simulink model "ControllerForOriginSensordata"  (R2017a)
settings: Solver=FixedStepAuto  StartTime=0.0  StopTime=10  FixedStep=dt  RelTol=1e-3
values from neighbouring files (symbols this model uses):
  dt = dtFC    [evalOriginSensordata.m]    (also in startControllerNL.m = 0.01)
  H_Drone = zeros(5,12)    [evalOriginSensordata.m]    (also in startControllerNL.m)
  H_TWB = zeros(3,12)    [evalOriginSensordata.m]    (also in startControllerNL.m)
  k1 = a    (= 1)    [evalOriginSensordata.m]    (also in startControllerNL.m)
  k10 = a    (= 1)    [evalOriginSensordata.m]    (also in startControllerNL.m)
  k11 = a    (= 1)    [evalOriginSensordata.m]    (also in startControllerNL.m)
  k12 = a    (= 1)    [evalOriginSensordata.m]    (also in startControllerNL.m)
  k2 = a    (= 1)    [evalOriginSensordata.m]    (also in startControllerNL.m)
  k3 = a    (= 1)    [evalOriginSensordata.m]    (also in startControllerNL.m)
  k4 = a    (= 1)    [evalOriginSensordata.m]    (also in startControllerNL.m)
  k5 = a    (= 1)    [evalOriginSensordata.m]    (also in startControllerNL.m)
  k6 = a    (= 1)    [evalOriginSensordata.m]    (also in startControllerNL.m)
  k7 = a    (= 1)    [evalOriginSensordata.m]    (also in startControllerNL.m)
  k8 = a    (= 1)    [evalOriginSensordata.m]    (also in startControllerNL.m)
  k9 = a    (= 1)    [evalOriginSensordata.m]    (also in startControllerNL.m)
  kd1 = d    (= 10)    [evalOriginSensordata.m]    (also in startControllerNL.m)
  kd2 = d    (= 10)    [evalOriginSensordata.m]    (also in startControllerNL.m)
  kd3 = d    (= 10)    [evalOriginSensordata.m]    (also in startControllerNL.m)
  kd4 = d    (= 10)    [evalOriginSensordata.m]    (also in startControllerNL.m)
  kp1 = p    (= 5)    [evalOriginSensordata.m]    (also in startControllerNL.m)
  kp2 = p    (= 5)    [evalOriginSensordata.m]    (also in startControllerNL.m)
  kp3 = p    (= 5)    [evalOriginSensordata.m]    (also in startControllerNL.m)
  kp4 = p    (= 5)    [evalOriginSensordata.m]    (also in startControllerNL.m)
  x_d = [sensordataTWB(end,[2:4]), 0]    [evalOriginSensordata.m]    (also in startControllerNL.m = [0 0 8 0])
libraries: simulink x2, sharedTrackingLibrary x1
settings Model: Creator=Schalker  LastModifiedBy=Schalker

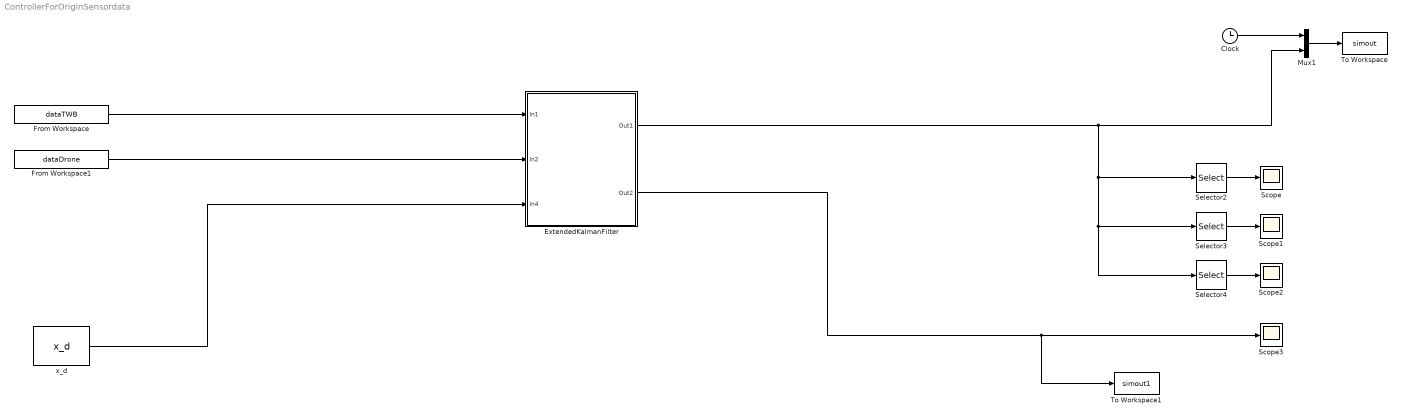
== system ControllerForOriginSensordata ==
  Clock : Clock
  "ExtendedKalmanFilter " : Subsystem
  From Workspace : FromWorkspace  VariableName=dataTWB  OutDataTypeStr=double  SampleTime=0
  From Workspace1 : FromWorkspace  VariableName=dataDrone  SampleTime=0
  Mux1 : Mux  Inputs=2
  Scope{,1..3} (4 alike) : Scope
  Selector2 : Selector  InputPortWidth=12  IndexOptions=Index vector (dialog)  Indices=1  OutputSizes=1
  Selector3 : Selector  InputPortWidth=12  IndexOptions=Index vector (dialog)  Indices=2  OutputSizes=1
  Selector4 : Selector  InputPortWidth=12  IndexOptions=Index vector (dialog)  Indices=3  OutputSizes=1
  To Workspace : ToWorkspace  VariableName=simout  SampleTime=-1
      settings: Save2DSignal=2-D array (concatenate along first dimension)
  To Workspace1 : ToWorkspace  VariableName=simout1  SampleTime=-1
      settings: Save2DSignal=2-D array (concatenate along first dimension)
  "x_d " : Constant  Value=x_d
  wires:
  Selector2/1 -> Scope/1
  Selector3/1 -> Scope1/1
  "ExtendedKalmanFilter "/1(Out1) -> Mux1/2, Selector4/1, Selector3/1, Selector2/1
  From Workspace/1 -> "ExtendedKalmanFilter "/1(In1)
  From Workspace1/1 -> "ExtendedKalmanFilter "/2(In2)
  "x_d "/1 -> "ExtendedKalmanFilter "/3(In4)
  "ExtendedKalmanFilter "/2(Out2) -> To Workspace1/1, Scope3/1
  Mux1/1 -> To Workspace/1
  Clock/1 -> Mux1/1
  Selector4/1 -> Scope2/1

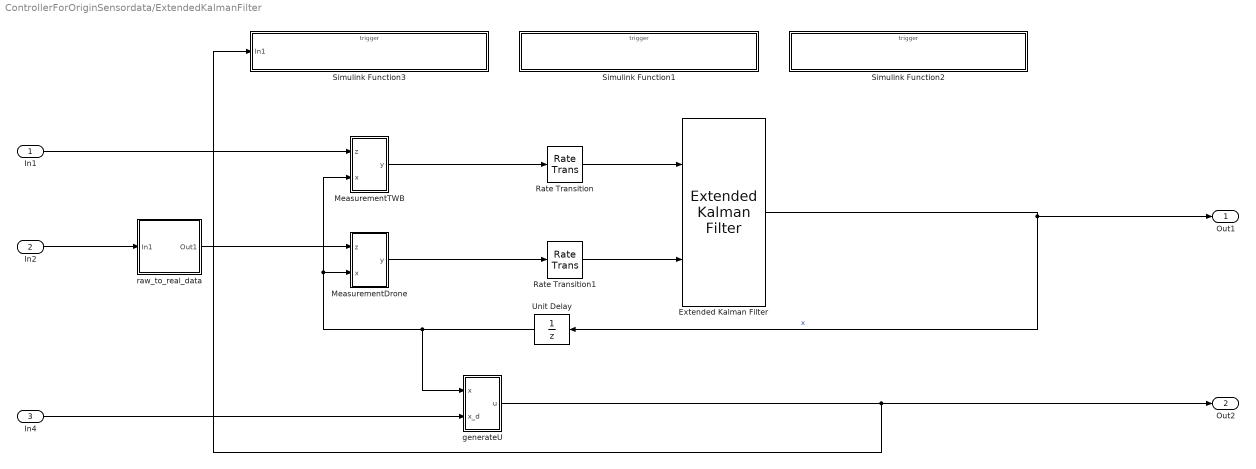
== system ControllerForOriginSensordata/ExtendedKalmanFilter  ==
  In1 : Inport
  In2 : Inport  Port=2
  In4 : Inport  Port=3
  Extended Kalman Filter : sharedTrackingLibrary/Extended Kalman Filter  StateTransitionFcn=stateTransitionFcn  HasStateTransitionJacobianFcn=off  HasAdditiveProcessNoise=Additive  ProcessNoise=processNoiseCovariance  HasTimeVaryingProcessNoise=off  HasStateTransitionFcnExtraArgument=0  InitialState=initialState  InitialStateCovariance=10  MeasurementFcn1=measurementTWBFcn  HasMeasurementJacobianFcn1=off  HasMeasurementEnablePort1=off  HasAdditiveMeasurementNoise1=Additive  MeasurementNoise1=measurementNoiseCovarianceTWB  HasTimeVaryingMeasurementNoise1=off  HasMeasurementFcnExtraArgument1=0  MeasurementFcn2=measurementDroneFcn  HasMeasurementJacobianFcn2=off  HasMeasurementEnablePort2=off  HasAdditiveMeasurementNoise2=Additive  MeasurementNoise2=measurementNoiseCovarianceDrone  HasTimeVaryingMeasurementNoise2=off  HasMeasurementFcnExtraArgument2=0  MeasurementFcn3=myMeasurementFcn  HasMeasurementJacobianFcn3=off  HasMeasurementEnablePort3=off  HasAdditiveMeasurementNoise3=Additive  MeasurementNoise3=1  HasTimeVaryingMeasurementNoise3=off  HasMeasurementFcnExtraArgument3=0  MeasurementFcn4=myMeasurementFcn  HasMeasurementJacobianFcn4=off  HasMeasurementEnablePort4=off  HasAdditiveMeasurementNoise4=Additive  MeasurementNoise4=1  HasTimeVaryingMeasurementNoise4=off  HasMeasurementFcnExtraArgument4=0  MeasurementFcn5=myMeasurementFcn  HasMeasurementJacobianFcn5=off  HasMeasurementEnablePort5=off  HasAdditiveMeasurementNoise5=Additive  MeasurementNoise5=1  HasTimeVaryingMeasurementNoise5=off  HasMeasurementFcnExtraArgument5=0  EnableMultirate=on  StateTransitionFcnSampleTime=dt  MeasurementFcn1SampleTime=dt  MeasurementFcn2SampleTime=dt  MeasurementFcn3SampleTime=1  MeasurementFcn4SampleTime=1  MeasurementFcn5SampleTime=1  UseCurrentEstimator=on  OutputStateCovariance=off  DataType=double  SampleTime=1  NumberOfMeasurements=2
  MeasurementDrone : Subsystem
  MeasurementTWB : Subsystem
  Rate Transition : RateTransition
  Rate Transition1 : RateTransition
  Simulink Function1 : Subsystem  TreatAsAtomicUnit=on
  Simulink Function2 : Subsystem  TreatAsAtomicUnit=on
  Simulink Function3 : Subsystem  TreatAsAtomicUnit=on
  Unit Delay : UnitDelay  SampleTime=-1
  generateU : Subsystem
  raw_to_real_data : Subsystem
  Out1 : Outport
  Out2 : Outport  Port=2
  wires:
  In1/1 -> MeasurementTWB/1(z)
  In4/1 -> generateU/2("x_d ")
  Extended Kalman Filter/1 -> Unit Delay/1, Out1/1  "x"
  MeasurementDrone/1(y) -> Rate Transition1/1
  Rate Transition1/1 -> Extended Kalman Filter/2
  In2/1 -> raw_to_real_data/1(In1)
  Rate Transition/1 -> Extended Kalman Filter/1
  Unit Delay/1 -> MeasurementDrone/2(x), MeasurementTWB/2(x), generateU/1(x)
  generateU/1(u) -> Out2/1, Simulink Function3/1(In1)
  MeasurementTWB/1(y) -> Rate Transition/1
  raw_to_real_data/1(Out1) -> MeasurementDrone/1(z)

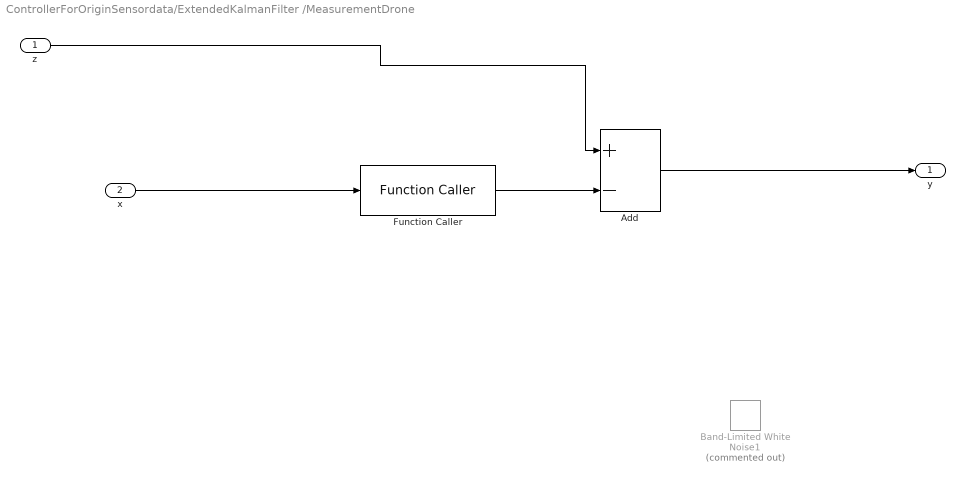
== system ControllerForOriginSensordata/ExtendedKalmanFilter /MeasurementDrone ==
  z : Inport
  x : Inport  Port=2
  Add : Sum  Inputs=+-
  Band-Limited White Noise1 : simulink/Sources/Band-Limited White Noise  Commented=on  Cov=5e-5  Ts=0.05  seed=[23341;23342]
  Function Caller : FunctionCaller  FunctionPrototype=y = measurementDroneFcn(x)
  y : Outport
  wires:
  Add/1 -> y/1
  z/1 -> Add/1
  Function Caller/1 -> Add/2
  x/1 -> Function Caller/1

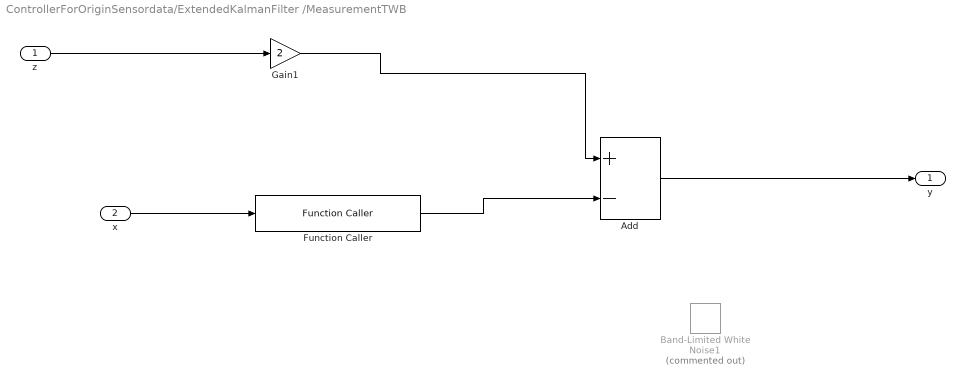
== system ControllerForOriginSensordata/ExtendedKalmanFilter /MeasurementTWB ==
  z : Inport
  x : Inport  Port=2
  Add : Sum  Inputs=+-
  Band-Limited White Noise1 : simulink/Sources/Band-Limited White Noise  Commented=on  Cov=5e-5  Ts=0.05  seed=[23341;23342]
  Function Caller : FunctionCaller  FunctionPrototype=y = measurementTWBFcn(x)
  Gain1 : Gain  Gain=2
  y : Outport
  wires:
  z/1 -> Gain1/1
  Add/1 -> y/1
  Function Caller/1 -> Add/2
  x/1 -> Function Caller/1
  Gain1/1 -> Add/1

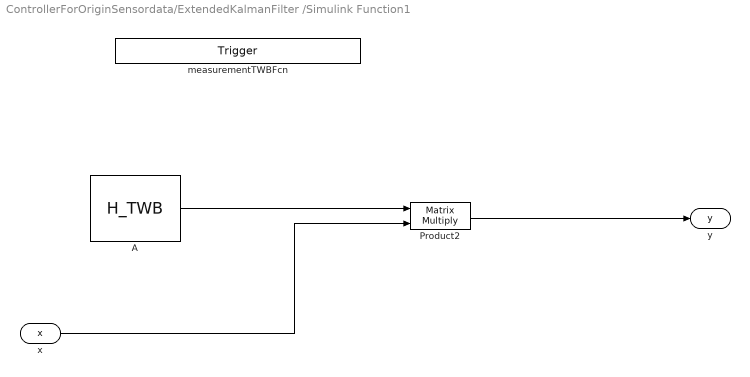
== system ControllerForOriginSensordata/ExtendedKalmanFilter /Simulink Function1 ==
  measurementTWBFcn : TriggerPort  TriggerType=function-call  IsSimulinkFunction=on  FunctionName=measurementTWBFcn  VariantControl=Variant
  A : Constant  Value=H_TWB
  Product2 : Product  Multiplication=Matrix(*)
  x : ArgIn  DisableCoverage=on  PortDimensions=12  ArgumentName=x
  y : ArgOut  DisableCoverage=on  PortDimensions=3  ArgumentName=y
  wires:
  A/1 -> Product2/1
  x/1 -> Product2/2
  Product2/1 -> y/1

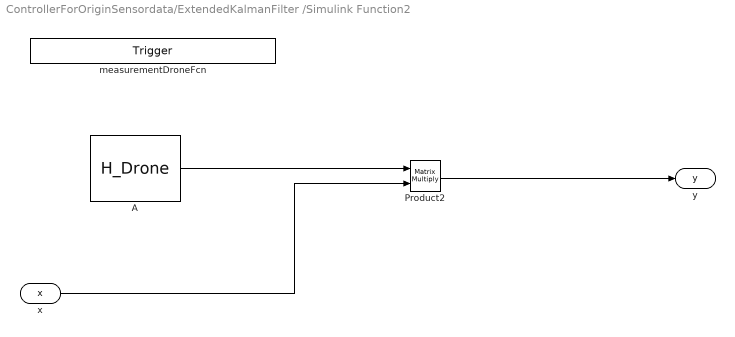
== system ControllerForOriginSensordata/ExtendedKalmanFilter /Simulink Function2 ==
  measurementDroneFcn : TriggerPort  TriggerType=function-call  IsSimulinkFunction=on  FunctionName=measurementDroneFcn  VariantControl=Variant
  A : Constant  Value=H_Drone
  Product2 : Product  Multiplication=Matrix(*)
  x : ArgIn  DisableCoverage=on  PortDimensions=12  ArgumentName=x
  y : ArgOut  DisableCoverage=on  PortDimensions=5  ArgumentName=y
  wires:
  Product2/1 -> y/1
  A/1 -> Product2/1
  x/1 -> Product2/2

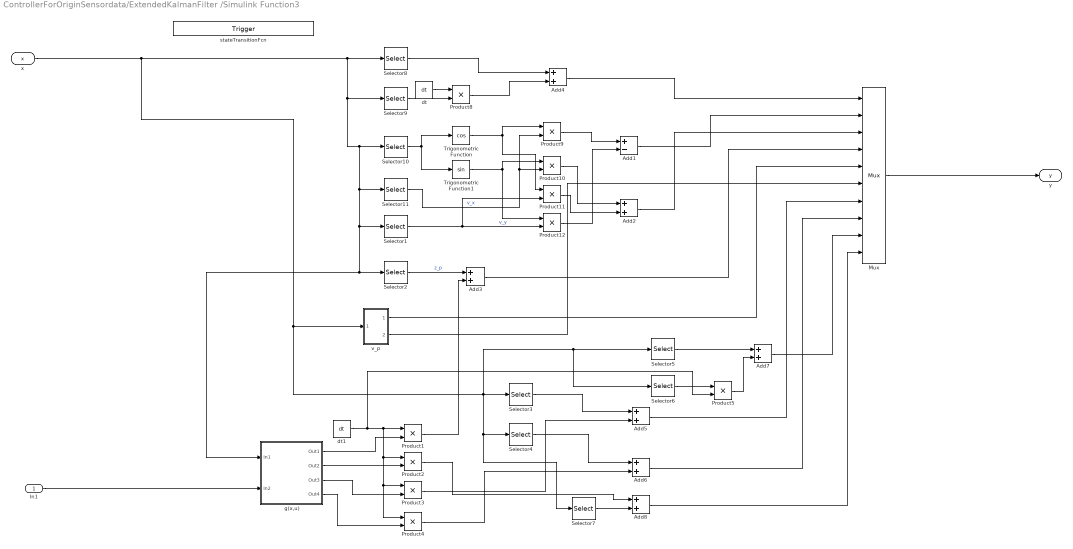
== system ControllerForOriginSensordata/ExtendedKalmanFilter /Simulink Function3 ==
  In1 : Inport
  stateTransitionFcn : TriggerPort  TriggerType=function-call  IsSimulinkFunction=on  FunctionName=stateTransitionFcn  VariantControl=Variant
  Add1 : Sum  Inputs=+-
  Add{2..8} (7 alike) : Sum
  Mux : Mux  Inputs=10
  Product{1..5,8..12} (10 alike) : Product
  Selector1 : Selector  InputPortWidth=12  IndexOptions=Index vector (dialog)  Indices=[8]  OutputSizes=1
  Selector10 : Selector  InputPortWidth=12  IndexOptions=Index vector (dialog)  Indices=[11]  OutputSizes=1
  Selector11 : Selector  InputPortWidth=12  IndexOptions=Index vector (dialog)  Indices=[7]  OutputSizes=1
  Selector2 : Selector  InputPortWidth=12  IndexOptions=Index vector (dialog)  Indices=[6]  OutputSizes=1
  Selector3 : Selector  InputPortWidth=12  IndexOptions=Index vector (dialog)  Indices=[9]  OutputSizes=1
  Selector4 : Selector  InputPortWidth=12  IndexOptions=Index vector (dialog)  Indices=[10]  OutputSizes=1
  Selector5 : Selector  InputPortWidth=12  IndexOptions=Index vector (dialog)  Indices=[11]  OutputSizes=1
  Selector6 : Selector  InputPortWidth=12  IndexOptions=Index vector (dialog)  Indices=[12]  OutputSizes=1
  Selector7 : Selector  InputPortWidth=12  IndexOptions=Index vector (dialog)  Indices=[12]  OutputSizes=1
  Selector8 : Selector  InputPortWidth=12  IndexOptions=Index vector (dialog)  Indices=[1 2 3]  OutputSizes=1
  Selector9 : Selector  InputPortWidth=12  IndexOptions=Index vector (dialog)  Indices=[4 5 6]  OutputSizes=1
  Trigonometric Function : Trigonometry  Operator=cos
  Trigonometric Function1 : Trigonometry
  dt : Constant  Value=dt
  dt1 : Constant  Value=dt
  g(x,u) : Subsystem
  v_p : Subsystem
  x : ArgIn  DisableCoverage=on  PortDimensions=12  ArgumentName=x
  y : ArgOut  DisableCoverage=on  PortDimensions=12  ArgumentName=y
  wires:
  x/1 -> Selector6/1, Selector5/1, Selector7/1, Selector4/1, Selector3/1, v_p/1(In1), Selector8/1, Selector11/1, Selector1/1, Selector2/1, g(x,u)/1(In1), Selector10/1, Selector9/1
  Selector9/1 -> Product8/2
  dt/1 -> Product8/1
  Product8/1 -> Add4/2
  Selector8/1 -> Add4/1
  Add4/1 -> Mux/1
  Selector10/1 -> Trigonometric Function1/1, Trigonometric Function/1
  Trigonometric Function/1 -> Product11/1, Product9/1
  Trigonometric Function1/1 -> Product12/1, Product10/1
  In1/1 -> g(x,u)/2(In2)
  Selector11/1 -> Product10/2, Product9/2  "v_x"
  Selector1/1 -> Product12/2, Product11/2  "v_y"
  Product9/1 -> Add1/1
  Product12/1 -> Add1/2
  Product10/1 -> Add2/1
  Product11/1 -> Add2/2
  Selector2/1 -> Add3/1  "z_p"
  g(x,u)/1(Out1) -> Product1/2
  Product1/1 -> Add3/2
  g(x,u)/2(Out2) -> Product2/2
  g(x,u)/3(Out3) -> Product3/2
  g(x,u)/4(Out4) -> Product4/2
  Add3/1 -> Mux/4
  v_p/1(Out1) -> Mux/5
  v_p/2(Out2) -> Mux/6
  Add1/1 -> Mux/2
  Add2/1 -> Mux/3
  Selector3/1 -> Add5/1
  Product3/1 -> Add5/2
  Selector4/1 -> Add6/1
  Product4/1 -> Add6/2
  Add5/1 -> Mux/7
  Add6/1 -> Mux/8
  Selector6/1 -> Product5/1
  dt1/1 -> Product5/2, Product2/1, Product4/1, Product3/1, Product1/1
  Selector5/1 -> Add7/1
  Product5/1 -> Add7/2
  Add7/1 -> Mux/9
  Selector7/1 -> Add8/2
  Product2/1 -> Add8/1
  Add8/1 -> Mux/10
  Mux/1 -> y/1

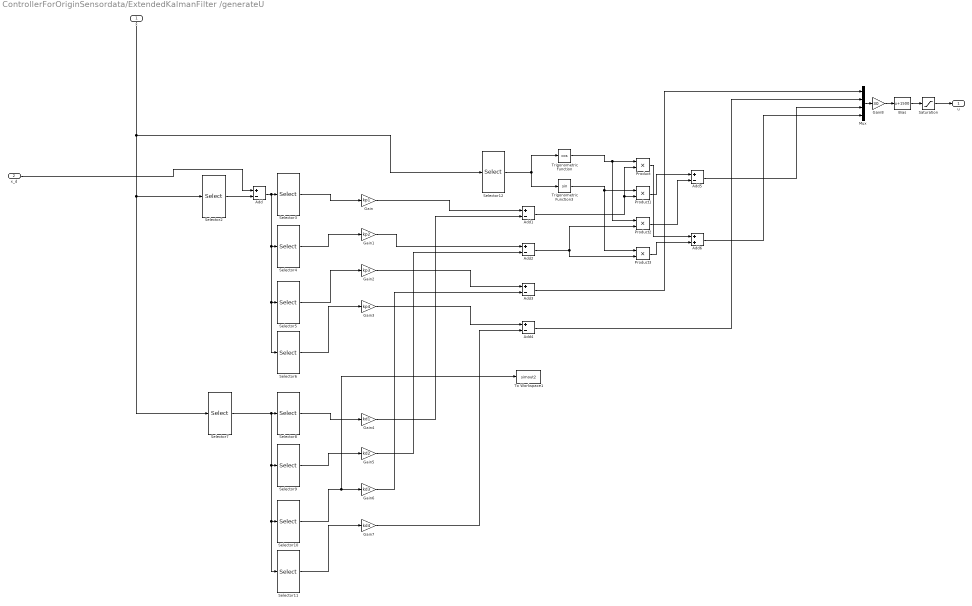
== system ControllerForOriginSensordata/ExtendedKalmanFilter /generateU ==
  x : Inport
  "x_d " : Inport  Port=2
  Add{,1..5} (6 alike) : Sum  Inputs=+-
  Add6 : Sum
  Bias : Bias  Bias=1500
  Gain : Gain  Gain=kp1
  Gain1 : Gain  Gain=kp2
  Gain2 : Gain  Gain=kp3
  Gain3 : Gain  Gain=kp4
  Gain4 : Gain  Gain=kd1
  Gain5 : Gain  Gain=kd2
  Gain6 : Gain  Gain=kd3
  Gain7 : Gain  Gain=kd4
  Gain8 : Gain  Gain=30
  Mux : Mux
  Product{,1..3} (4 alike) : Product
  Saturation : Saturate  UpperLimit=3000  LowerLimit=0
  Selector10 : Selector  InputPortWidth=4  IndexOptions=Index vector (dialog)  Indices=3  OutputSizes=1
  Selector11 : Selector  InputPortWidth=4  IndexOptions=Index vector (dialog)  Indices=4  OutputSizes=1
  Selector12 : Selector  InputPortWidth=12  IndexOptions=Index vector (dialog)  Indices=11  OutputSizes=1
  Selector2 : Selector  InputPortWidth=12  IndexOptions=Index vector (dialog)  Indices=[1 2 3 11]  OutputSizes=1
  Selector3 : Selector  InputPortWidth=4  IndexOptions=Index vector (dialog)  Indices=[1]  OutputSizes=1
  Selector4 : Selector  InputPortWidth=4  IndexOptions=Index vector (dialog)  Indices=2  OutputSizes=1
  Selector5 : Selector  InputPortWidth=4  IndexOptions=Index vector (dialog)  Indices=3  OutputSizes=1
  Selector6 : Selector  InputPortWidth=4  IndexOptions=Index vector (dialog)  Indices=4  OutputSizes=1
  Selector7 : Selector  InputPortWidth=12  IndexOptions=Index vector (dialog)  Indices=[4 5 6 12]  OutputSizes=1
  Selector8 : Selector  InputPortWidth=4  IndexOptions=Index vector (dialog)  Indices=[1]  OutputSizes=1
  Selector9 : Selector  InputPortWidth=4  IndexOptions=Index vector (dialog)  Indices=2  OutputSizes=1
  To Workspace1 : ToWorkspace  VariableName=simout2  SampleTime=-1
      settings: Save2DSignal=2-D array (concatenate along first dimension)
  Trigonometric Function : Trigonometry  Operator=cos
  Trigonometric Function3 : Trigonometry
  u : Outport
  wires:
  Selector3/1 -> Gain/1
  "x_d "/1 -> Add/1
  Gain1/1 -> Add2/1
  Product2/1 -> Add5/2
  Add2/1 -> Product3/2, Product2/2
  Selector4/1 -> Gain1/1
  Add4/1 -> Mux/2
  Selector2/1 -> Add/2
  Add6/1 -> Mux/4
  Add5/1 -> Mux/3
  Product1/1 -> Add5/1
  Gain/1 -> Add1/1
  Selector6/1 -> Gain3/1
  Gain7/1 -> Add4/2
  Add3/1 -> Mux/1
  Selector11/1 -> Gain7/1
  Selector7/1 -> Selector8/1, Selector9/1, Selector10/1, Selector11/1
  Selector10/1 -> To Workspace1/1, Gain6/1
  Selector9/1 -> Gain5/1
  Selector8/1 -> Gain4/1
  Gain6/1 -> Add3/2
  Gain3/1 -> Add4/1
  Add1/1 -> Product1/2, Product/2
  Selector12/1 -> Trigonometric Function/1, Trigonometric Function3/1
  Add/1 -> Selector6/1, Selector5/1, Selector4/1, Selector3/1
  Gain4/1 -> Add1/2
  x/1 -> Selector12/1, Selector7/1, Selector2/1
  Gain2/1 -> Add3/1
  Product3/1 -> Add6/2
  Product/1 -> Add6/1
  Trigonometric Function/1 -> Product2/1, Product/1
  Trigonometric Function3/1 -> Product3/1, Product1/1
  Gain5/1 -> Add2/2
  Selector5/1 -> Gain2/1
  Mux/1 -> Gain8/1
  Bias/1 -> Saturation/1
  Gain8/1 -> Bias/1
  Saturation/1 -> u/1

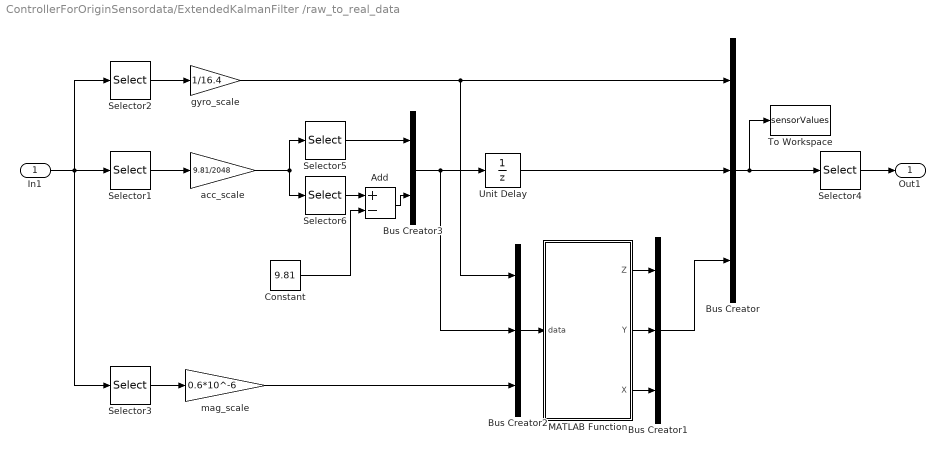
== system ControllerForOriginSensordata/ExtendedKalmanFilter /raw_to_real_data ==
  In1 : Inport  PortDimensions=11
  Add : Sum  Inputs=+-
  Bus Creator : BusCreator  Inputs=3
  Bus Creator1 : BusCreator  Inputs=3
  Bus Creator2 : BusCreator  Inputs=3
  Bus Creator3 : BusCreator  Inputs=2
  Constant : Constant  Value=9.81
  MATLAB Function : MATLAB Function  TreatAsAtomicUnit=on
  Selector1 : Selector  InputPortWidth=11  IndexOptions=Index vector (dialog)  Indices=[4,5,6]  OutputSizes=1
  Selector2 : Selector  InputPortWidth=11  IndexOptions=Index vector (dialog)  Indices=[1,2,3]  OutputSizes=1
  Selector3 : Selector  InputPortWidth=11  IndexOptions=Index vector (dialog)  Indices=[1:9]  OutputSizes=1
  Selector4 : Selector  InputPortWidth=9  IndexOptions=Index vector (dialog)  Indices=[4,5,7,8,9]  OutputSizes=1
  Selector5 : Selector  InputPortWidth=3  IndexOptions=Index vector (dialog)  Indices=[1,2]  OutputSizes=1
  Selector6 : Selector  InputPortWidth=3  IndexOptions=Index vector (dialog)  Indices=3  OutputSizes=1
  To Workspace : ToWorkspace  VariableName=sensorValues  SampleTime=-1
      settings: Save2DSignal=2-D array (concatenate along first dimension)
  Unit Delay : UnitDelay  SampleTime=-1
  acc_scale : Gain  Gain=9.81/2048
  gyro_scale : Gain  Gain=1/16.4
  mag_scale : Gain  Gain=0.6*10^-6
  Out1 : Outport  PortDimensions=5
  wires:
  In1/1 -> Selector3/1, Selector1/1, Selector2/1
  MATLAB Function/1(Z) -> Bus Creator1/1
  Selector2/1 -> gyro_scale/1
  Selector1/1 -> acc_scale/1
  gyro_scale/1 -> Bus Creator2/1, Bus Creator/1
  Selector3/1 -> mag_scale/1
  MATLAB Function/2(Y) -> Bus Creator1/2
  MATLAB Function/3(X) -> Bus Creator1/3
  Selector4/1 -> Out1/1
  acc_scale/1 -> Selector6/1, Selector5/1
  mag_scale/1 -> Bus Creator2/3
  Bus Creator2/1 -> MATLAB Function/1(data)
  Bus Creator/1 -> To Workspace/1, Selector4/1
  Bus Creator1/1 -> Bus Creator/3
  Selector6/1 -> Add/1
  Selector5/1 -> Bus Creator3/1
  Add/1 -> Bus Creator3/2
  Constant/1 -> Add/2
  Bus Creator3/1 -> Bus Creator2/2, Unit Delay/1
  Unit Delay/1 -> Bus Creator/2

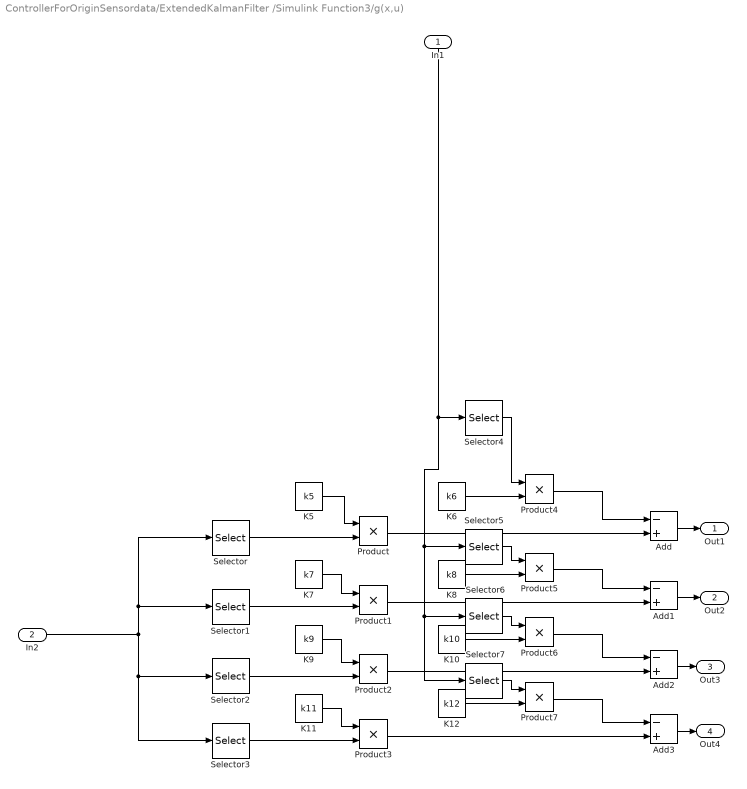
== system ControllerForOriginSensordata/ExtendedKalmanFilter /Simulink Function3/g(x,u) ==
  In1 : Inport
  In2 : Inport  Port=2
  Add{,1..3} (4 alike) : Sum  Inputs=-+
  K10 : Constant  Value=k10
  K11 : Constant  Value=k11
  K12 : Constant  Value=k12
  K5 : Constant  Value=k5
  K6 : Constant  Value=k6
  K7 : Constant  Value=k7
  K8 : Constant  Value=k8
  K9 : Constant  Value=k9
  Product{,1..7} (8 alike) : Product
  Selector : Selector  InputPortWidth=4  IndexOptions=Index vector (dialog)  Indices=[1]  OutputSizes=1
  Selector1 : Selector  InputPortWidth=4  IndexOptions=Index vector (dialog)  Indices=[2]  OutputSizes=1
  Selector2 : Selector  InputPortWidth=4  IndexOptions=Index vector (dialog)  Indices=[3]  OutputSizes=1
  Selector3 : Selector  InputPortWidth=4  IndexOptions=Index vector (dialog)  Indices=[4]  OutputSizes=1
  Selector4 : Selector  InputPortWidth=12  IndexOptions=Index vector (dialog)  Indices=[6]  OutputSizes=1
  Selector5 : Selector  InputPortWidth=12  IndexOptions=Index vector (dialog)  Indices=[12]  OutputSizes=1
  Selector6 : Selector  InputPortWidth=12  IndexOptions=Index vector (dialog)  Indices=[9]  OutputSizes=1
  Selector7 : Selector  InputPortWidth=12  IndexOptions=Index vector (dialog)  Indices=[10]  OutputSizes=1
  Out1 : Outport
  Out2 : Outport  Port=2
  Out3 : Outport  Port=3
  Out4 : Outport  Port=4
  wires:
  K7/1 -> Product1/1
  Selector6/1 -> Product6/1
  Selector2/1 -> Product2/2
  Product/1 -> Add/2
  Product6/1 -> Add2/1
  Selector/1 -> Product/2
  Add2/1 -> Out3/1
  In1/1 -> Selector7/1, Selector6/1, Selector5/1, Selector4/1
  Add3/1 -> Out4/1
  Add/1 -> Out1/1
  Add1/1 -> Out2/1
  K9/1 -> Product2/1
  Selector4/1 -> Product4/1
  In2/1 -> Selector/1, Selector1/1, Selector3/1, Selector2/1
  Product2/1 -> Add2/2
  K8/1 -> Product5/2
  Product3/1 -> Add3/2
  Product1/1 -> Add1/2
  Selector5/1 -> Product5/1
  Product5/1 -> Add1/1
  Selector3/1 -> Product3/2
  K5/1 -> Product/1
  K12/1 -> Product7/2
  Product7/1 -> Add3/1
  K10/1 -> Product6/2
  Product4/1 -> Add/1
  Selector1/1 -> Product1/2
  Selector7/1 -> Product7/1
  K11/1 -> Product3/1
  K6/1 -> Product4/2

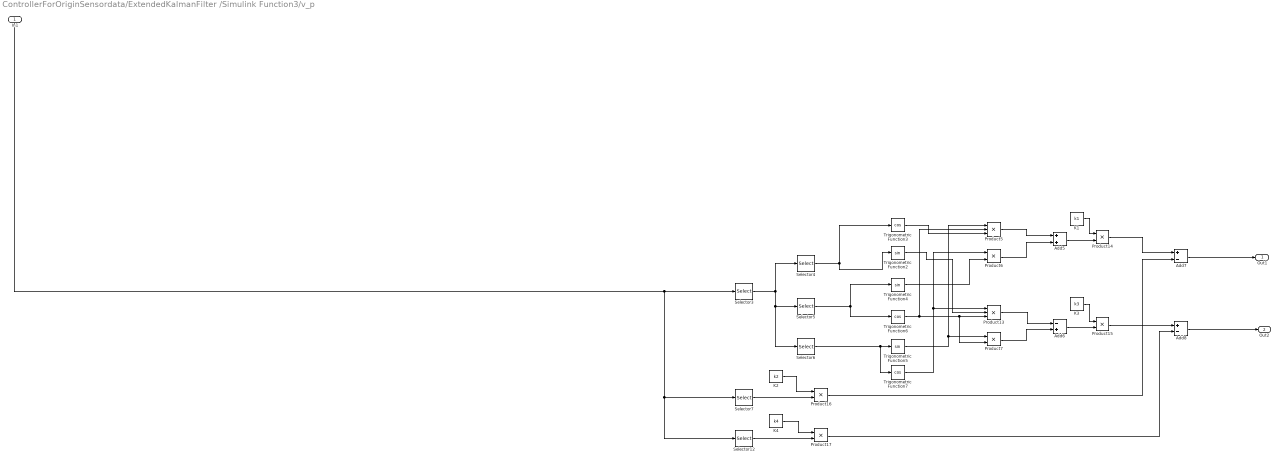
== system ControllerForOriginSensordata/ExtendedKalmanFilter /Simulink Function3/v_p ==
  In1 : Inport
  Add5 : Sum
  Add6 : Sum  Inputs=-+
  Add7 : Sum  Inputs=+-
  Add8 : Sum  Inputs=+-
  K1 : Constant  Value=k1
  K2 : Constant  Value=k2
  K3 : Constant  Value=k3
  K4 : Constant  Value=k4
  Product13 : Product  Inputs=3
  Product{6..7,14..17} (6 alike) : Product
  Product5 : Product  Inputs=3
  Selector12 : Selector  InputPortWidth=12  IndexOptions=Index vector (dialog)  Indices=[8]  OutputSizes=1
  Selector3 : Selector  InputPortWidth=12  IndexOptions=Index vector (dialog)  Indices=[9 10 11]  OutputSizes=1
  Selector4 : Selector  InputPortWidth=3  IndexOptions=Index vector (dialog)  Indices=[1]  OutputSizes=1
  Selector5 : Selector  InputPortWidth=3  IndexOptions=Index vector (dialog)  Indices=[2]  OutputSizes=1
  Selector6 : Selector  InputPortWidth=3  IndexOptions=Index vector (dialog)  Indices=[3]  OutputSizes=1
  Selector7 : Selector  InputPortWidth=12  IndexOptions=Index vector (dialog)  Indices=[7]  OutputSizes=1
  Trigonometric Function2 : Trigonometry
  Trigonometric Function3 : Trigonometry  Operator=cos
  Trigonometric Function4 : Trigonometry
  Trigonometric Function5 : Trigonometry
  Trigonometric Function6 : Trigonometry  Operator=cos
  Trigonometric Function7 : Trigonometry  Operator=cos
  Out1 : Outport
  Out2 : Outport  Port=2
  wires:
  In1/1 -> Selector12/1, Selector7/1, Selector3/1
  Selector6/1 -> Trigonometric Function5/1, Trigonometric Function7/1
  Trigonometric Function4/1 -> Product6/2
  Product6/1 -> Add5/2
  Add7/1 -> Out1/1
  Add5/1 -> Product14/2
  K1/1 -> Product14/1
  Product13/1 -> Add6/1
  Product16/1 -> Add7/2
  Product17/1 -> Add8/2
  Trigonometric Function6/1 -> Product7/2, Product13/3, Product5/2
  K2/1 -> Product16/1
  Selector5/1 -> Trigonometric Function6/1, Trigonometric Function4/1
  Trigonometric Function2/1 -> Product13/2
  Add8/1 -> Out2/1
  Selector7/1 -> Product16/2
  Product14/1 -> Add7/1
  Trigonometric Function5/1 -> Product5/1, Product7/1
  Product5/1 -> Add5/1
  Selector12/1 -> Product17/2
  Selector4/1 -> Trigonometric Function3/1, Trigonometric Function2/1
  Selector3/1 -> Selector6/1, Selector5/1, Selector4/1
  Product7/1 -> Add6/2
  Product15/1 -> Add8/1
  Add6/1 -> Product15/2
  Trigonometric Function7/1 -> Product13/1, Product6/1
  Trigonometric Function3/1 -> Product5/3
  K4/1 -> Product17/1
  K3/1 -> Product15/1

== matlab function ControllerForOriginSensordata/ExtendedKalmanFilter /raw_to_real_data/MATLAB Function ==
  data: data input; Z output; Y output; X output
function [Z,Y,X] = fcn(data)
    %% Process sensor data through algorithm
    data = data';
    gyroscope = data(1,[1:3]);
    accelerometer = data(1,[4:6]);
    magnetometer = data(1,[7:9]);
    AHRS = MadgwickAHRS('SamplePeriod', 1/256, 'Beta', 0.1);
    % AHRS = MahonyAHRS('SamplePeriod', 1/256, 'Kp', 0.5);

    quaternion = zeros(1, 4);
    AHRS.Update(gyroscope(1,:) * (pi/180), accelerometer(1,:), magnetometer(1,:));	% gyroscope units must be radians
    quaternion = AHRS.Quaternion;

    euler = quatern2euler(quaternConj(quaternion));	% use conjugate for sensor frame relative to Earth. Unit is rad.
    Z = euler(1,1);
    Y = euler(1,2);
    X = euler(1,3);

end

% function obj = MadgwickAHRS(varargin)
%     for i = 1:2:nargin
%         if  strcmp(varargin{i}, 'SamplePeriod'), obj.SamplePeriod = varargin{i+1};
%         elseif  strcmp(varargin{i}, 'Quaternion'), obj.Quaternion = varargin{i+1};
%         elseif  strcmp(varargin{i}, 'Beta'), obj.Beta = varargin{i+1};
%         else error('Invalid argument');
%         end
%     end;
% end
% function obj = Update(obj, Gyroscope, Accelerometer, Magnetometer)
%     q = obj.Quaternion; % short name local variable for readability
% 
%     % Normalise accelerometer measurement
%     if(norm(Accelerometer) == 0), return; end	% handle NaN
%     Accelerometer = Accelerometer / norm(Accelerometer);	% normalise magnitude
% 
%     % Normalise magnetometer measurement
%     if(norm(Magnetometer) == 0), return; end	% handle NaN
%     Magnetometer = Magnetometer / norm(Magnetometer);	% normalise magnitude
% 
%     % Reference direction of Earth's magnetic feild
%     h = quaternProd(q, quaternProd([0 Magnetometer], quaternConj(q)));
%     b = [0 norm([h(2) h(3)]) 0 h(4)];
% 
%     % Gradient decent algorithm corrective step
%     F = [2*(q(2)*q(4) - q(1)*q(3)) - Accelerometer(1)
%         2*(q(1)*q(2) + q(3)*q(4)) - Accelerometer(2)
%         2*(0.5 - q(2)^2 - q(3)^2) - Accelerometer(3)
%         2*b(2)*(0.5 - q(3)^2 - q(4)^2) + 2*b(4)*(q(2)*q(4) - q(1)*q(3)) - Magnetometer(1)
%         2*b(2)*(q(2)*q(3) - q(1)*q(4)) + 2*b(4)*(q(1)*q(2) + q(3)*q(4)) - Magnetometer(2)
%         2*b(2)*(q(1)*q(3) + q(2)*q(4)) + 2*b(4)*(0.5 - q(2)^2 - q(3)^2) - Magnetometer(3)];
%     J = [-2*q(3),                 	2*q(4),                    -2*q(1),                         2*q(2)
%         2*q(2),                 	2*q(1),                    	2*q(4),                         2*q(3)
%         0,                         -4*q(2),                    -4*q(3),                         0
%         -2*b(4)*q(3),               2*b(4)*q(4),               -4*b(2)*q(3)-2*b(4)*q(1),       -4*b(2)*q(4)+2*b(4)*q(2)
%         -2*b(2)*q(4)+2*b(4)*q(2),	2*b(2)*q(3)+2*b(4)*q(1),	2*b(2)*q(2)+2*b(4)*q(4),       -2*b(2)*q(1)+2*b(4)*q(3)
%         2*b(2)*q(3),                2*b(2)*q(4)-4*b(4)*q(2),	2*b(2)*q(1)-4*b(4)*q(3),        2*b(2)*q(2)];
%     step = (J'*F);
%     step = step / norm(step);	% normalise step magnitude
% 
%     % Compute rate of change of quaternion
%     qDot = 0.5 * quaternProd(q, [0 Gyroscope(1) Gyroscope(2) Gyroscope(3)]) - obj.Beta * step';
% 
%     % Integrate to yield quaternion
%     q = q + qDot * obj.SamplePeriod;
%     obj.Quaternion = q / norm(q); % normalise quaternion
% end
% 
% function obj = UpdateIMU(obj, Gyroscope, Accelerometer)
%     q = obj.Quaternion; % short name local variable for readability
% 
%     % Normalise accelerometer measurement
%     if(norm(Accelerometer) == 0), return; end	% handle NaN
%     Accelerometer = Accelerometer / norm(Accelerometer);	% normalise magnitude
% 
%     % Gradient decent algorithm corrective step
%     F = [2*(q(2)*q(4) - q(1)*q(3)) - Accelerometer(1)
%         2*(q(1)*q(2) + q(3)*q(4)) - Accelerometer(2)
%         2*(0.5 - q(2)^2 - q(3)^2) - Accelerometer(3)];
%     J = [-2*q(3),	2*q(4),    -2*q(1),	2*q(2)
%         2*q(2),     2*q(1),     2*q(4),	2*q(3)
%         0,         -4*q(2),    -4*q(3),	0    ];
%     step = (J'*F);
%     step = step / norm(step);	% normalise step magnitude
% 
%     % Compute rate of change of quaternion
%     qDot = 0.5 * quaternProd(q, [0 Gyroscope(1) Gyroscope(2) Gyroscope(3)]) - obj.Beta * step';
% 
%     % Integrate to yield quaternion
%     q = q + qDot * obj.SamplePeriod;
%     obj.Quaternion = q / norm(q); % normalise quaternion
% end
